simulink model "foc"  (R2021b)
settings: Solver=FixedStepDiscrete  StartTime=0.0  StopTime=20  FixedStep=Ts  MaxStep=1e-4  RelTol=1e-3
model workspace (MAT data in the model file):
  flux = 0.154
values from neighbouring files (symbols this model uses):
  currt_width = 200.0    [motor_parameters.sldd]
  Flux = 0.00103001    [motor_parameters.sldd]
  Ibus = 5.0    [motor_parameters.sldd]
  Ld = 2.235E-5    [motor_parameters.sldd]
  Lq = 2.567E-5    [motor_parameters.sldd]
  Ls = 2.235E-5    [motor_parameters.sldd]
  OPL_time = 3.0    [motor_parameters.sldd]
  Pn = 7.0    [motor_parameters.sldd]
  R = 0.083    [motor_parameters.sldd]
  Rs = 0.112    [motor_parameters.sldd]
  smo_l = 0.1    [motor_parameters.sldd]
  smo_m = 0.001    [motor_parameters.sldd]
  Ts = 0.0001    [motor_parameters.sldd]
  Ubus = 12.0    [motor_parameters.sldd]
undefined symbols (not defined in the file or in its folder): DiscIntNeverNeededParam, sigbuilder_block, spd_ki, spd_kp
libraries: slpidlib x5, simulink x3, mcbcontrolslib x3, mcbplantlib x1, autolibpmsmexterior x1
(part 1 of 2)
settings Model: DataDictionary=motor_parameters.sldd  Creator=chenpeng  LastModifiedBy=chenpeng
settings OptimizationCC: DefaultParameterBehavior=Inlined  UseDivisionForNetSlopeComputation=on  GainParamInheritBuiltInType=on  UseFloatMulNetSlope=on  InlineInvariantSignals=on  PassReuseOutputArgsAs=Individual arguments  ZeroExternalMemoryAtStartup=off  ZeroInternalMemoryAtStartup=off  NoFixptDivByZeroProtection=on  EfficientFloat2IntCast=on  LifeSpan=1  OptimizeBlockOrder=speed  DifferentSizesBufferReuse=on  EfficientTunableParamExpr=on
settings DebuggingCC: AlgebraicLoopMsg=none  ParameterTunabilityLossMsg=error
settings HardwareCC: ProdBitPerPointer=32  ProdBitPerSizeT=32  ProdBitPerPtrDiffT=32  ProdLargestAtomicInteger=Long  ProdLargestAtomicFloat=Double  ProdWordSize=32  ProdLongLongMode=on  ProdHWDeviceType=ARM Compatible->ARM Cortex-M
settings SFSimCC: MATLABDynamicMemAlloc=off
settings RTWCC: Description=Embedded Coder  SystemTargetFile=ert.tlc  GenCodeOnly=on  TemplateMakefile=ert_default_tmf  Toolchain=GNU Tools for ARM Embedded Processors
settings CodeAppCC: ForceParamTrailComments=on  IgnoreCustomStorageClasses=off  OperatorAnnotations=on  SimulinkDataObjDesc=on  SFDataObjDesc=on  CustomSymbolStrGlobalVar=rt$N$M  CustomSymbolStrType=$N$M  CustomSymbolStrFcn=$N$M$F  CustomSymbolStrMacro=$N$M  InsertBlockDesc=on
settings ERTTargetCC: TargetLangStandard=C99 (ISO)  GenerateSampleERTMain=on  IncludeMdlTerminateFcn=off  CombineSignalStateStructs=on  SupportComplex=off  SupportNonInlinedSFcns=on  InlinedParameterPlacement=NonHierarchical  ERTCustomFileTemplate=example_file_process.tlc  ERTFilePackagingFormat=CompactWithDataFile

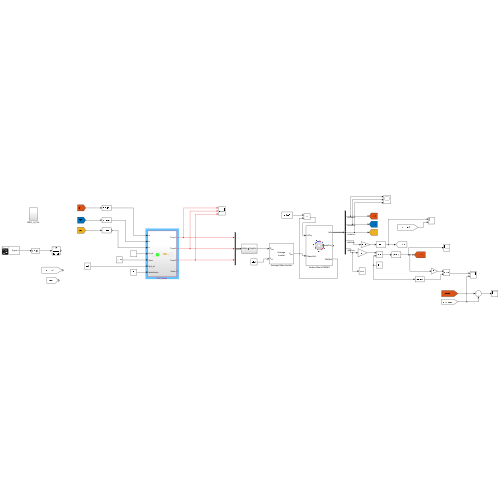
[thumbnail: Simulink's stored preview of the top-level diagram]
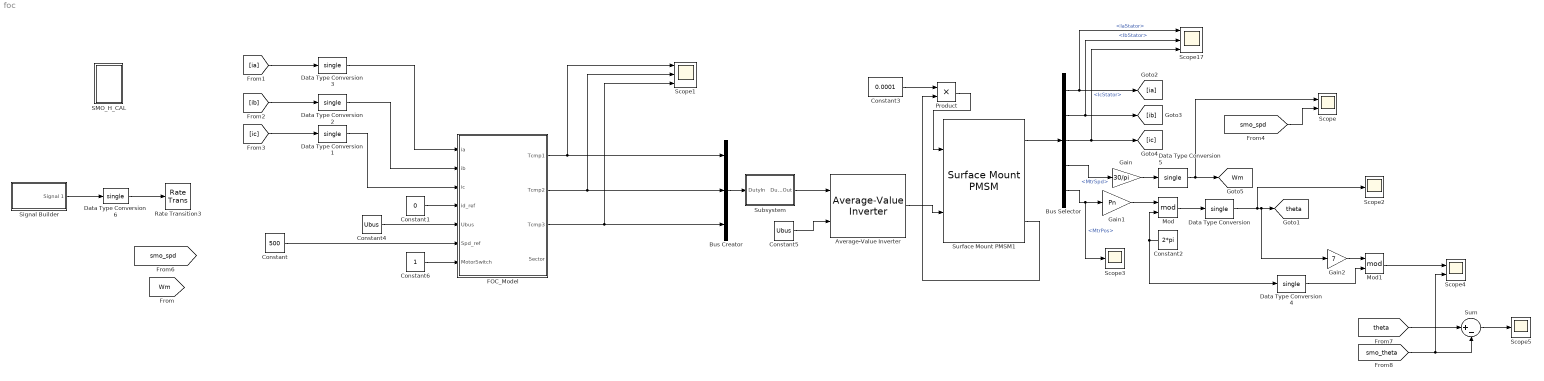
== system foc ==
  Average-Value Inverter : mcbplantlib/Average-Value Inverter
  Bus Creator : BusCreator  Inputs=3
  Bus Selector : BusSelector  OutputSignals=IaStator,IbStator,IcStator,MtrSpd,MtrPos
  Constant : Constant  Value=500  OutDataTypeStr=single  SampleTime=-1
  Constant1 : Constant  Value=0  OutDataTypeStr=single  SampleTime=-1
  Constant2 : Constant  Value=2*pi
  Constant3 : Constant  Value=0.0001  OutDataTypeStr=double
  Constant4 : Constant  Value=Ubus  OutDataTypeStr=single
  Constant5 : Constant  Value=Ubus  OutDataTypeStr=single
  Constant6 : Constant  OutDataTypeStr=single  SampleTime=-1
  Data Type Conversion{,1..6} (7 alike) : DataTypeConversion  OutDataTypeStr=single
  FOC_Model : Subsystem
  Gain : Gain  Gain=30/pi
  Gain1 : Gain  Gain=Pn
  Gain2 : Gain  Gain=7
  Mod : Math  Operator=mod  SaturateOnIntegerOverflow=on
  Mod1 : Math  Operator=mod  SaturateOnIntegerOverflow=on
  Product : Product
  Rate Transition3 : RateTransition
  SMO_H_CAL : Subsystem
  Scope : Scope  NumInputPorts=2
  Scope1 : Scope  NumInputPorts=3
  Scope17 : Scope  NumInputPorts=3
  Scope2 : Scope
  Scope3 : Scope
  Scope4 : Scope  NumInputPorts=2
  Scope5 : Scope
  Signal Builder : Subsystem  Tag=STV Subsys  LoadFcn=sigbuilder_block('load');  StartFcn=sigbuilder_block('start');  StopFcn=sigbuilder_block('stop');  ClipboardFcn=sigbuilder_block('clipboard');  mask(Sigbuilder block){tuvar=[0:10]}
      mask help: Simulink:masks:SigbuilderBlock_MD
      mask init:
      | if ~strcmp(get_param(bdroot(gcbh),'SimulationStatus'),'stopped') tuvar = sigbuilder_block('maskInit'); end
      settings: CopyFcn=sigbuilder_block('copy');  DeleteFcn=sigbuilder_block('delete');  ModelCloseFcn=sigbuilder_block('modelClose');  PreSaveFcn=sigbuilder_block('preSave');  PauseFcn=sigbuilder_block('pause');  ContinueFcn=sigbuilder_block('continue');  NameChangeFcn=sigbuilder_block('namechange');  OpenFcn=sigbuilder_block('open',[437.6 199.2 550.4 400 ]);  CloseFcn=sigbuilder_block('close');
      mask Display: plot(0, 0, 100, 100,[2, 2, 32, 32, 2], [68, 8, 8, 68, 68],[32, 2], [38, 38], [32, 19, 2],[53, 60, 44], [32, 17, 17, 2],[16, 16, 31, 31]);txt = getActiveGroup(gcbh);text(2, 100, txt,'verticalAlignment', 'top');
  Subsystem : Subsystem
  Sum : Sum  Inputs=|+-
  Surface Mount PMSM1 : autolibpmsmexterior/Surface Mount PMSM  port_config=Torque  sim_type=Discrete  Ts=Ts  FilePath=E:\Sandbox\Bauto\Work\surfacepmsm_motordata.m  P=Pn  Rs=Rs  Ldq_=Ls  KConstText=Permanent flux linkage constant (lambda_pm):  lambda_pm=Flux  Ke=159.9771  Kt=1.323  mechanical=[0.0027, 4.924e-4, 0]  idq0=[0 0]  theta_init=0  omega_init=0  KConst=Flux  lambda_pm_calc=Flux  RefBlkName='autolibpmsmexterior/Surface Mount PMSM'  aMode=1  Ldq="[0.0003752   0.0003752]"
      settings: SourceProductBaseCode=PW,DR,MT,UV,VE
  tag scope: Wm=global, theta=global
  wires:
  Data Type Conversion/1 -> Scope2/1, Gain2/1, [theta]
  Bus Selector/3 -> Scope17/3, [ic]  "<IcStator>"
  Mod/1 -> Data Type Conversion/1
  Gain/1 -> Data Type Conversion5/1
  Constant3/1 -> Product/1
  Gain1/1 -> Mod/1
  Data Type Conversion5/1 -> Scope/1, [Wm]
  Bus Creator/1 -> Subsystem/1(DutyIn)
  Bus Selector/5 -> Scope3/1, Gain1/1  "<MtrPos>"
  Bus Selector/1 -> [ia], Scope17/1  "<IaStator>"
  Subsystem/1(DutyOut) -> Average-Value Inverter/1
  Bus Selector/2 -> Scope17/2, [ib]  "<IbStator>"
  Bus Selector/4 -> Gain/1  "<MtrSpd>"
  Constant2/1 -> Data Type Conversion4/1, Mod/2
  Constant5/1 -> Average-Value Inverter/2
  [ia] -> Data Type Conversion3/1
  [ib] -> Data Type Conversion2/1
  [ic] -> Data Type Conversion1/1
  Average-Value Inverter/1 -> Surface Mount PMSM1/2
  Surface Mount PMSM1/3 -> Product/2
  Surface Mount PMSM1/1 -> Bus Selector/1
  Gain2/1 -> Mod1/1
  Mod1/1 -> Scope4/1
  Data Type Conversion4/1 -> Mod1/2
  Product/1 -> Surface Mount PMSM1/1
  Data Type Conversion3/1 -> FOC_Model/1(ia)
  Data Type Conversion2/1 -> FOC_Model/2(ib)
  Data Type Conversion1/1 -> FOC_Model/3(ic)
  Constant4/1 -> FOC_Model/5(Ubus)
  FOC_Model/1(Tcmp1) -> Scope1/1, Bus Creator/1
  FOC_Model/2(Tcmp2) -> Scope1/2, Bus Creator/2
  FOC_Model/3(Tcmp3) -> Scope1/3, Bus Creator/3
  Constant6/1 -> FOC_Model/7(MotorSwitch)
  [smo_spd] -> Scope/2
  Constant1/1 -> FOC_Model/4(id_ref)
  [smo_theta] -> Scope4/2, Sum/2
  Sum/1 -> Scope5/1
  Data Type Conversion6/1 -> Rate Transition3/1
  Signal Builder/1(Signal 1) -> Data Type Conversion6/1
  Constant/1 -> FOC_Model/6(Spd_ref)
  [theta] -> Sum/1

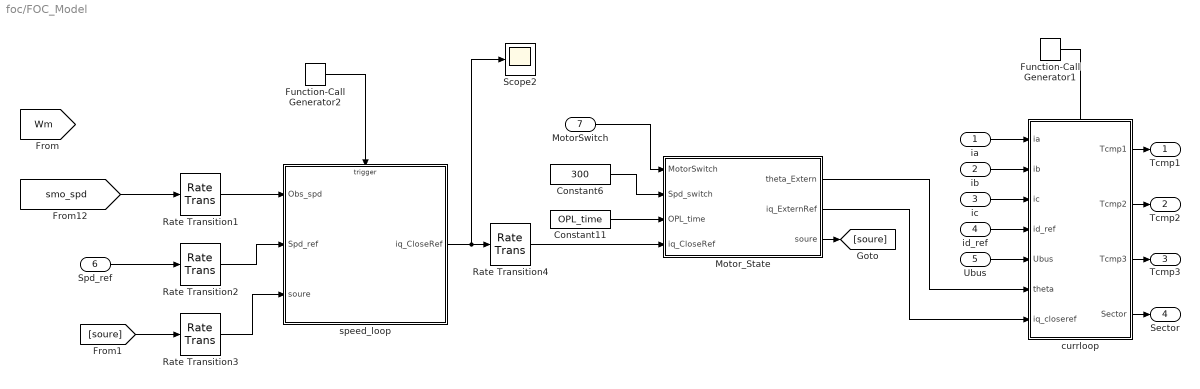
== system foc/FOC_Model ==
  ia : Inport  OutDataTypeStr=single
  ib : Inport  Port=2  OutDataTypeStr=single
  ic : Inport  Port=3  OutDataTypeStr=single
  id_ref : Inport  Port=4  OutDataTypeStr=single
  Ubus : Inport  Port=5  OutDataTypeStr=single
  Spd_ref : Inport  Port=6  OutDataTypeStr=single
  MotorSwitch : Inport  Port=7  OutDataTypeStr=single
  Constant11 : Constant  Value=OPL_time  OutDataTypeStr=single
  Constant6 : Constant  Value=300  OutDataTypeStr=int32
  Function-Call Generator1 : simulink/Ports & Subsystems/Function-Call Generator  sample_time=1e-4  numberOfIterations=1  DisallowWideOutput=off
  Function-Call Generator2 : simulink/Ports & Subsystems/Function-Call Generator  sample_time=1e-3  numberOfIterations=1  DisallowWideOutput=off
  Motor_State : Subsystem
  Rate Transition{1..4} (4 alike) : RateTransition
  Scope2 : Scope
  currloop : Subsystem
  speed_loop : Subsystem  TreatAsAtomicUnit=on  SystemSampleTime=1e-4
      settings: RTWSystemCode=Nonreusable function  RTWFcnNameOpts=Use subsystem name
  Tcmp1 : Outport  OutDataTypeStr=single
  Tcmp2 : Outport  Port=2  OutDataTypeStr=single
  Tcmp3 : Outport  Port=3  OutDataTypeStr=single
  Sector : Outport  Port=4  OutDataTypeStr=single
  wires:
  Rate Transition1/1 -> speed_loop/1(Obs_spd)
  ia/1 -> currloop/1(ia)
  ib/1 -> currloop/2(ib)
  Ubus/1 -> currloop/5(Ubus)
  currloop/4(Sector) -> Sector/1
  currloop/2(Tcmp2) -> Tcmp2/1
  Rate Transition2/1 -> speed_loop/2(Spd_ref)
  speed_loop/1(iq_CloseRef) -> Scope2/1, Rate Transition4/1
  ic/1 -> currloop/3(ic)
  id_ref/1 -> currloop/4(id_ref)
  currloop/1(Tcmp1) -> Tcmp1/1
  currloop/3(Tcmp3) -> Tcmp3/1
  Spd_ref/1 -> Rate Transition2/1
  Constant11/1 -> Motor_State/3(OPL_time)
  Rate Transition4/1 -> Motor_State/4(iq_CloseRef)
  Constant6/1 -> Motor_State/2(Spd_switch)
  MotorSwitch/1 -> Motor_State/1(MotorSwitch)
  Motor_State/1(theta_Extern) -> currloop/6(theta)
  Motor_State/2(iq_ExternRef) -> currloop/7(iq_closeref)
  Function-Call Generator1/1 -> ?
  Rate Transition3/1 -> speed_loop/3(soure)
  Function-Call Generator2/1 -> speed_loop/Trigger
  Motor_State/3(soure) -> [soure]
  [soure] -> Rate Transition3/1
  [smo_spd] -> Rate Transition1/1

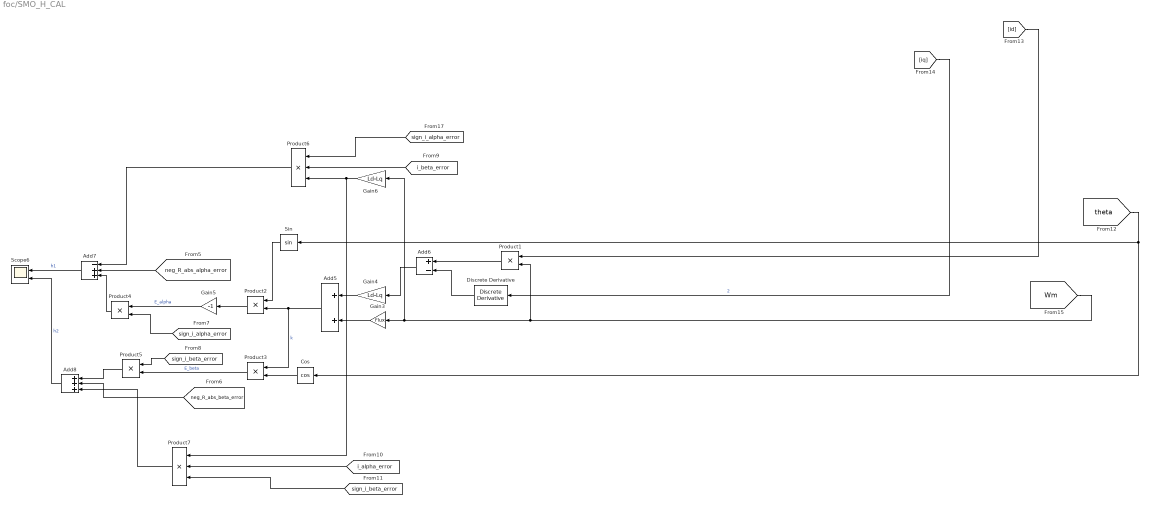
== system foc/SMO_H_CAL ==
  Add5 : Sum
  Add6 : Sum  Inputs=+-
  Add7 : Sum  Inputs=-++  AccumDataTypeStr=single
  Add8 : Sum  Inputs=+++
  Cos : Trigonometry  Operator=cos
  Discrete Derivative : simulink/Discrete/Discrete Derivative  gainval=1.0  ICPrevScaledInput=0.0  OutMin=[]  OutMax=[]  OutDataType=fixdt(1, 16)  OutScaling=2^-10  DoSatur=off
  Gain3 : Gain  Gain=Flux
  Gain4 : Gain  Gain=Ld-Lq
  Gain5 : Gain  Gain=-1
  Gain6 : Gain  Gain=Ld-Lq
  Product{1..5} (5 alike) : Product
  Product6 : Product  Inputs=3  OutDataTypeStr=single
  Product7 : Product  Inputs=3
  Scope6 : Scope  NumInputPorts=2
  Sin : Trigonometry
  wires:
  Add5/1 -> Product3/1, Product2/2  "k"
  [sign_i_beta_error] -> Product7/3
  Cos/1 -> Product3/2
  [neg_R_abs_beta_error] -> Add8/2
  Gain6/1 -> Product6/3, Product7/1
  [sign_i_alpha_error] -> Product4/2
  [theta] -> Cos/1, Sin/1
  [iq] -> Discrete Derivative/1  "2"
  Product1/1 -> Add6/1
  [Wm] -> Gain6/1, Gain3/1, Product1/2
  [sign_i_alpha_error] -> Product6/1
  Product6/1 -> Add7/1
  [neg_R_abs_alpha_error] -> Add7/2
  Product4/1 -> Add7/3
  Product2/1 -> Gain5/1
  [i_alpha_error] -> Product7/2
  Gain4/1 -> Add5/1
  Discrete Derivative/1 -> Add6/2
  Add7/1 -> Scope6/1  "h1"
  [id] -> Product1/1
  [i_beta_error] -> Product6/2
  Gain5/1 -> Product4/1  "E_alpha"
  Product3/1 -> Product5/2  "E_beta"
  Product7/1 -> Add8/3
  Add6/1 -> Gain4/1
  Add8/1 -> Scope6/2  "h2"
  Gain3/1 -> Add5/2
  [sign_i_beta_error] -> Product5/1
  Sin/1 -> Product2/1
  Product5/1 -> Add8/1

== system foc/Signal Builder ==
  Demux : Demux  Tag=STV Demux  Outputs=1
      settings: DisplayOption=none
  FromWs : FromWorkspace  Tag=STV FromWs  VariableName=tuvar
      SigBuilderData=|
      | common.afterFinalStr = 'Extrapolate'
      | common.sampleTime = 0
      | dataSet.timeRange = [0 10]
      | dataSet.name = 'Group 1'
      | sbobj.Groups.Name = 'Group 1'
      | sbobj.Groups.Signals.Name = 'Signal 1'
      | sbobj.Groups.Signals.XData = [0 4 4 7 7 10]
      | sbobj.Groups.Signals.YData = [400 395 598 602 800 802]
  Signal 1 : Outport  Tag=STV Outport
  wires:
  Demux/1 -> Signal 1/1
  FromWs/1 -> Demux/1

== system foc/Subsystem ==
  DutyIn : Inport
  Constant : Constant  Value=0.5  OutDataTypeStr=double  SampleTime=-1
  Gain : Gain  Gain=1/8000  ParamDataTypeStr=single
  Gain1 : Gain  Gain=-1
  Sum : Sum  Inputs=|+-
  Sum1 : Sum  Inputs=|++
  DutyOut : Outport
  wires:
  Sum/1 -> Gain1/1
  Constant/1 -> Sum1/2, Sum/2
  DutyIn/1 -> Gain/1
  Gain1/1 -> Sum1/1
  Sum1/1 -> DutyOut/1
  Gain/1 -> Sum/1

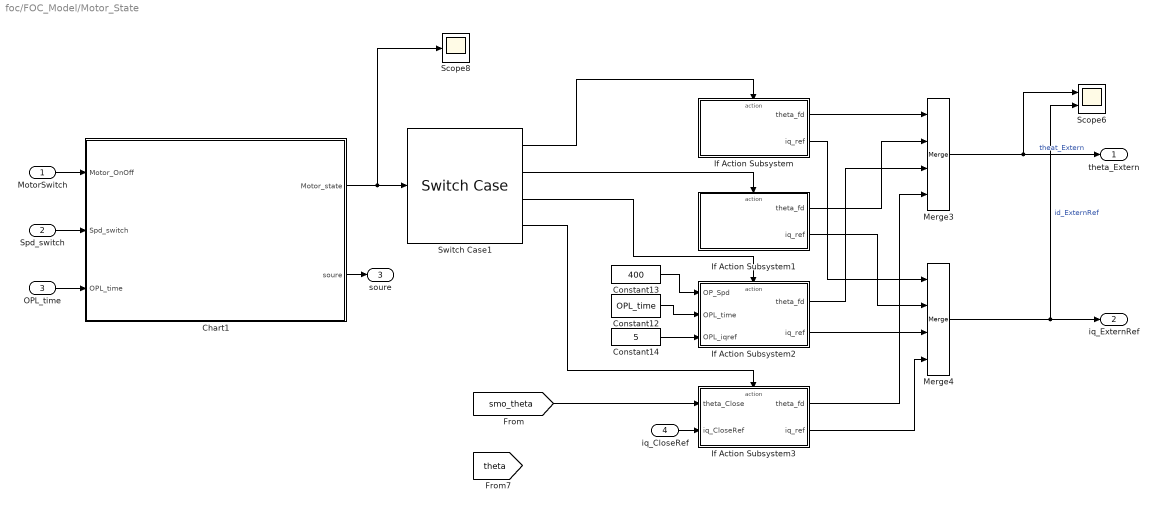
== system foc/FOC_Model/Motor_State ==
  MotorSwitch : Inport
  Spd_switch : Inport  Port=2  OutDataTypeStr=int32
  OPL_time : Inport  Port=3  OutDataTypeStr=single
  iq_CloseRef : Inport  Port=4
  Chart1 : Stateflow chart  TreatAsAtomicUnit=on
  Constant12 : Constant  Value=OPL_time  OutDataTypeStr=single
  Constant13 : Constant  Value=400  OutDataTypeStr=int32
  Constant14 : Constant  Value=5  OutDataTypeStr=single
  If Action Subsystem : Subsystem  TreatAsAtomicUnit=on
  If Action Subsystem1 : Subsystem  TreatAsAtomicUnit=on
  If Action Subsystem2 : Subsystem  TreatAsAtomicUnit=on
  If Action Subsystem3 : Subsystem  TreatAsAtomicUnit=on
  Merge3 : Merge  Inputs=4
  Merge4 : Merge  Inputs=4
  Scope6 : Scope  NumInputPorts=2
  Scope8 : Scope
  Switch Case1 : SwitchCase  CaseConditions={1,2,3,4}  ShowDefaultCase=off
  theta_Extern : Outport  OutDataTypeStr=single
  iq_ExternRef : Outport  Port=2  OutDataTypeStr=single
  soure : Outport  Port=3
  wires:
  Constant13/1 -> If Action Subsystem2/1(OP_Spd)
  Constant14/1 -> If Action Subsystem2/3(OPL_iqref)
  Constant12/1 -> If Action Subsystem2/2(OPL_time)
  iq_CloseRef/1 -> If Action Subsystem3/2(iq_CloseRef)
  Switch Case1/4 -> If Action Subsystem3/Action
  If Action Subsystem/1(theta_fd) -> Merge3/1
  Chart1/2(soure) -> soure/1
  OPL_time/1 -> Chart1/3(OPL_time)
  Merge4/1 -> iq_ExternRef/1, Scope6/2  "id_ExternRef"
  Spd_switch/1 -> Chart1/2(Spd_switch)
  Merge3/1 -> Scope6/1, theta_Extern/1  "theat_Extern"
  If Action Subsystem1/2(iq_ref) -> Merge4/2
  Chart1/1(Motor_state) -> Switch Case1/1, Scope8/1
  If Action Subsystem/2(iq_ref) -> Merge4/1
  Switch Case1/2 -> If Action Subsystem1/Action
  Switch Case1/1 -> If Action Subsystem/Action
  If Action Subsystem3/1(theta_fd) -> Merge3/4
  Switch Case1/3 -> If Action Subsystem2/Action
  If Action Subsystem2/2(iq_ref) -> Merge4/3
  If Action Subsystem3/2(iq_ref) -> Merge4/4
  MotorSwitch/1 -> Chart1/1(Motor_OnOff)
  If Action Subsystem2/1(theta_fd) -> Merge3/3
  If Action Subsystem1/1(theta_fd) -> Merge3/2
  [smo_theta] -> If Action Subsystem3/1(theta_Close)

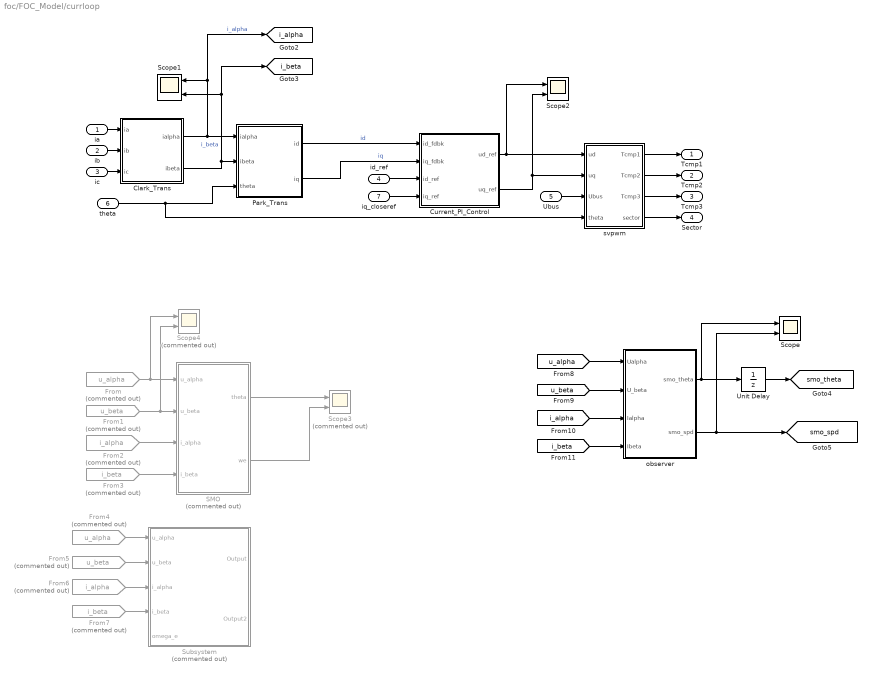
== system foc/FOC_Model/currloop ==
  ia : Inport  OutDataTypeStr=single  SampleTime=0.0001
  ib : Inport  Port=2  OutDataTypeStr=single  SampleTime=0.0001
  ic : Inport  Port=3  OutDataTypeStr=single  SampleTime=0.0001
  id_ref : Inport  Port=4  OutDataTypeStr=single  SampleTime=0.0001
  Ubus : Inport  Port=5  SampleTime=0.0001
  theta : Inport  Port=6  OutDataTypeStr=single  SampleTime=0.0001
  iq_closeref : Inport  Port=7  OutDataTypeStr=single  SampleTime=0.0001
  Clark_Trans : Subsystem  TreatAsAtomicUnit=on
  Current_PI_Control : Subsystem
  From : From  Commented=on  GotoTag=u_alpha  TagVisibility=global
  From1 : From  Commented=on  GotoTag=u_beta  TagVisibility=global
  From2 : From  Commented=on  GotoTag=i_alpha  TagVisibility=global
  From3 : From  Commented=on  GotoTag=i_beta  TagVisibility=global
  From4 : From  Commented=on  GotoTag=u_alpha  TagVisibility=global
  From5 : From  Commented=on  GotoTag=u_beta  TagVisibility=global
  From6 : From  Commented=on  GotoTag=i_alpha  TagVisibility=global
  From7 : From  Commented=on  GotoTag=i_beta  TagVisibility=global
  Park_Trans : Subsystem  TreatAsAtomicUnit=on
  SMO : Subsystem  Commented=on
      settings: PortSchema="{\"entries\":[{\"content\":{\"sides\":[{\"content\":{\"connectorIds\":[\"Out1\",\"Out2\"]},\"type\":\"ConnectorPlacement.EquallySpacedRectSide\",\"uuid\":\"5414e755-aa17-4597-a468-b801bf68950d\"},{\"content\":{\"connectorIds\":[\"In1\",\"In2\",\"In3\",\"In4\"],\"side\":\"RIGHT\"},\"type\":\"ConnectorPlacement.EquallySpacedRectSide\",\"uuid\":\"33e6150f-a627-4b89-8f54-9d41cb10a0e9\"},{\"content\":{\"connectorIds\":[],\"side\":\"TOP\"},\"type\":\"ConnectorPlacement.EquallySpacedRectSide\",\"uuid\":\"8ba45070-0913-41de-bd30-b153cef900e1\"}]},\"type\":\"ConnectorPlacement.EquallySpacedConnector\",\"uuid\":\"5336ec09-c709-45c9-9606-7ae9e0652068\"}],\"packageUris\":[\"http://schema.mathworks.com/mf0/Connector/R2020b\"],\"version\":\"1.0\"}"
  Scope : Scope  NumInputPorts=2
  Scope1 : Scope  NumInputPorts=2
  Scope2 : Scope  NumInputPorts=2
  Scope3 : Scope  Commented=on  NumInputPorts=2
  Scope4 : Scope  Commented=on  NumInputPorts=2
  Subsystem : Subsystem  Commented=on
  Unit Delay : UnitDelay  SampleTime=-1  HasFrameUpgradeWarning=on
  observer : Subsystem
  svpwm : Subsystem
  Tcmp1 : Outport
  Tcmp2 : Outport  Port=2
  Tcmp3 : Outport  Port=3
  Sector : Outport  Port=4
  tag scope: i_alpha=global, i_beta=global, smo_spd=global, smo_theta=global
  wires:
  Park_Trans/2(iq) -> Current_PI_Control/2(iq_fdbk)  "iq"
  ia/1 -> Clark_Trans/1(ia)
  ic/1 -> Clark_Trans/3(ic)
  Park_Trans/1(id) -> Current_PI_Control/1(id_fdbk)  "id"
  ib/1 -> Clark_Trans/2(ib)
  Current_PI_Control/1(ud_ref) -> Scope2/1, svpwm/1(ud)
  Current_PI_Control/2(uq_ref) -> Scope2/2, svpwm/2(uq)
  svpwm/1(Tcmp1) -> Tcmp1/1
  svpwm/2(Tcmp2) -> Tcmp2/1
  svpwm/3(Tcmp3) -> Tcmp3/1
  svpwm/4(sector) -> Sector/1
  Ubus/1 -> svpwm/3(Ubus)
  id_ref/1 -> Current_PI_Control/3(id_ref)
  From/1 -> Scope4/1, SMO/1(u_alpha)
  From1/1 -> Scope4/2, SMO/2(u_beta)
  From2/1 -> SMO/3(i_alpha)
  From3/1 -> SMO/4(i_beta)
  SMO/1(theta) -> Scope3/1
  SMO/2(we) -> Scope3/2
  Clark_Trans/2(ibeta) -> [i_beta], Scope1/2, Park_Trans/2(ibeta)  "i_beta"
  Clark_Trans/1(ialpha) -> [i_alpha], Scope1/1, Park_Trans/1(ialpha)  "i_alpha"
  From4/1 -> Subsystem/1(u_alpha)
  From7/1 -> Subsystem/4(i_beta)
  From6/1 -> Subsystem/3(i_alpha)
  From5/1 -> Subsystem/2(u_beta)
  theta/1 -> svpwm/4(theta), Park_Trans/3(theta)
  iq_closeref/1 -> Current_PI_Control/4(iq_ref)
  [u_alpha] -> observer/1(Ualpha)
  observer/1(smo_theta) -> Unit Delay/1, Scope/1
  observer/2(smo_spd) -> [smo_spd], Scope/2
  [i_beta] -> observer/4(Ibeta)
  [u_beta] -> observer/2(U_beta)
  [i_alpha] -> observer/3(Ialpha)
  Unit Delay/1 -> [smo_theta]

== system foc/FOC_Model/speed_loop ==
  Obs_spd : Inport  OutDataTypeStr=single  PortDimensions=1
  Spd_ref : Inport  Port=2  OutDataTypeStr=single  PortDimensions=1
  soure : Inport  Port=3  OutDataTypeStr=single  PortDimensions=1
  Trigger : TriggerPort  TriggerType=function-call  VariantControl=(inherit)  PortDimensions=1
  Constant : Constant  Value=0.0144  OutDataTypeStr=single  SampleTime=-1
  Constant1 : Constant  Value=0.6389  OutDataTypeStr=single  SampleTime=-1
  PID Controller3 : slpidlib/PID Controller  Controller=PI  Form=Parallel  TimeDomain=Discrete-time  UseExternalTs=off  SampleTime=-1  IntegratorMethod=Forward Euler  FilterMethod=Forward Euler  ControllerParametersSource=external  P=spd_kp  I=spd_ki  D=0  UseFilter=on  N=100  TunerSelectOption=Transfer Function Based (PID Tuner App)  InitialConditionSource=internal  InitialConditionForIntegrator=0  InitialConditionForFilter=0  DifferentiatorICPrevScaledInput=0  ExternalReset=rising  TrackingMode=off  Kt=1  LimitOutput=on  SatLimitsSource=internal  UpperSaturationLimit=Ibus  LowerSaturationLimit=-Ibus  LinearizeAsGain=on  AntiWindupMode=clamping  Kb=0.013  PGainOutDataTypeStr=single  PProdOutDataTypeStr=single  POutMin=[]  POutMax=[]  IGainOutDataTypeStr=single  IProdOutDataTypeStr=single  IOutMin=[]  IOutMax=[]  DOutMin=[]  DOutMax=[]  NOutMin=[]  NOutMax=[]  SumOutDataTypeStr=single  SumOutMin=[]  SumOutMax=[]  SaturationOutDataTypeStr=single  SaturationOutMin=[]  SaturationOutMax=[]  PParamMin=[]  PParamMax=[]  IParamMin=[]  IParamMax=[]  DParamMin=[]  DParamMax=[]  NParamMin=[]  NParamMax=[]  KbParamMin=[]  KbParamMax=[]  KtParamMin=[]  KtParamMax=[]  KbOutMin=[]  KbOutMax=[]  KtOutMin=[]  KtOutMax=[]  IntegratorOutMin=[]  IntegratorOutMax=[]  FilterOutMin=[]  FilterOutMax=[]  SumI1OutMin=[]  SumI1OutMax=[]  SumI2OutMin=[]  SumI2OutMax=[]  SumI3OutMin=[]  SumI3OutMax=[]  SumI4OutMin=[]  SumI4OutMax=[]  SumDOutMin=[]  SumDOutMax=[]  DifferentiatorOutMin=[]  DifferentiatorOutMax=[]  FilterDiffOutCoefMin=[]  FilterDiffOutCoefMax=[]  ReciprocalOutMin=[]  ReciprocalOutMax=[]  SumDenOutMin=[]  SumDenOutMax=[]  SumNumOutMin=[]  SumNumOutMax=[]  DivideOutMin=[]  DivideOutMax=[]  UdiffTsProdOutMin=[]  UdiffTsProdOutMax=[]  NTsProdOutMin=[]  NTsProdOutMax=[]  UintegralTsProdOutMin=[]  UintegralTsProdOutMax=[]  UngainTsProdOutMin=[]  UngainTsProdOutMax=[]  IntegratorContinuousStateAttributes=''  IntegratorStateMustResolveToSignalObject=off  IntegratorRTWStateStorageClass=Auto  FilterContinuousStateAttributes=''  FilterStateMustResolveToSignalObject=off  FilterRTWStateStorageClass=Auto  ParallelPVariant=ExternalParameters  IdealPVariant=Disabled  IVariant=ExternalParameters  DVariant=Disabled  IntegratorVariant=Discrete  SatVariant=Enabled  AWVariant=DiscClampingParallel  PCopyVariant=Disabled  TRVariant=Disabled  FdbkBlocksVariant=Forward  IdealPFdbkVariant=Disabled  SatFdbkVariant=Disabled  DerivativeFilterVariant=Disabled  NVariant=Disabled  NCopyVariant=Disabled_SignalSpec  FilterICVariant=Disabled  IntegratorICVariant=InternalICs  ExternalResetVariant=ExternalReset  TRSumVariant=Passthrough  SumFdbkVariant=Disabled  SumVariant=Sum_PI  TsampFilterVariant=InternalTs  TsampNgainVariant=Passthrough  TsampIntegralVariant=Passthrough  ExternalSaturationOutDataTypeStr=single
  Scope : Scope
  Sum2 : Sum  Inputs=|+-  AccumDataTypeStr=single  OutDataTypeStr=single
  iq_CloseRef : Outport
  wires:
  Obs_spd/1 -> Sum2/2
  Spd_ref/1 -> Sum2/1
  Sum2/1 -> Scope/1, PID Controller3/1
  PID Controller3/1 -> iq_CloseRef/1
  Constant/1 -> PID Controller3/2
  Constant1/1 -> PID Controller3/3
  soure/1 -> PID Controller3/4

== system foc/FOC_Model/Motor_State/If Action Subsystem ==
  Action Port : ActionPort  ActionPortLabel=case [ 1 ]:
  Constant : Constant  Value=0  OutDataTypeStr=single  SampleTime=-1
  Constant1 : Constant  Value=0  OutDataTypeStr=single  SampleTime=-1
  theta_fd : Outport
  iq_ref : Outport  Port=2
  wires:
  Constant/1 -> theta_fd/1
  Constant1/1 -> iq_ref/1

== system foc/FOC_Model/Motor_State/If Action Subsystem1 ==
  Action Port : ActionPort  ActionPortLabel=case [ 2 ]:
  Constant : Constant  Value=0  OutDataTypeStr=single  SampleTime=-1
  Constant1 : Constant  Value=2  OutDataTypeStr=single  SampleTime=-1
  theta_fd : Outport
  iq_ref : Outport  Port=2
  wires:
  Constant/1 -> theta_fd/1
  Constant1/1 -> iq_ref/1

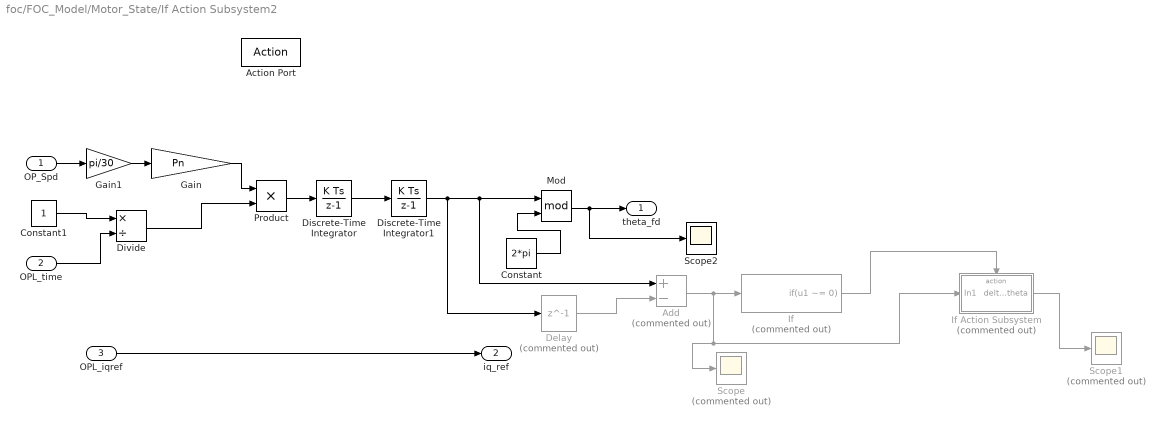
== system foc/FOC_Model/Motor_State/If Action Subsystem2 ==
  OP_Spd : Inport  OutDataTypeStr=int32  PortDimensions=1
  OPL_time : Inport  Port=2  OutDataTypeStr=single  PortDimensions=1
  OPL_iqref : Inport  Port=3  OutDataTypeStr=single  PortDimensions=1
  Action Port : ActionPort  ActionPortLabel=case [ 3 ]:
  Add : Sum  Commented=on  Inputs=+-  AccumDataTypeStr=single  OutDataTypeStr=single
  Constant : Constant  Value=2*pi  OutDataTypeStr=single  SampleTime=-1
  Constant1 : Constant  OutDataTypeStr=single  SampleTime=-1
  Delay : Delay  Commented=on  DelayLength=1  InputProcessing=Columns as channels (frame based)
  Discrete-Time Integrator : DiscreteIntegrator  SampleTime=-1  ICPrevOutput=DiscIntNeverNeededParam  ICPrevScaledInput=DiscIntNeverNeededParam
  Discrete-Time Integrator1 : DiscreteIntegrator  SampleTime=-1  ICPrevOutput=DiscIntNeverNeededParam  ICPrevScaledInput=DiscIntNeverNeededParam
  Divide : Product  Inputs=*/  OutDataTypeStr=single
  Gain : Gain  Gain=Pn
  Gain1 : Gain  Gain=pi/30  OutDataTypeStr=single
  If : If  Commented=on  IfExpression=u1 ~= 0  ShowElse=off
  If Action Subsystem : Subsystem  Commented=on  TreatAsAtomicUnit=on
  Mod : Math  Operator=mod  SaturateOnIntegerOverflow=on
  Product : Product  OutDataTypeStr=single
  Scope : Scope  Commented=on
  Scope1 : Scope  Commented=on
  Scope2 : Scope
  theta_fd : Outport
  iq_ref : Outport  Port=2
  wires:
  Gain1/1 -> Gain/1
  Constant1/1 -> Divide/1
  Gain/1 -> Product/1
  Discrete-Time Integrator/1 -> Discrete-Time Integrator1/1
  Constant/1 -> Mod/2
  Discrete-Time Integrator1/1 -> Delay/1, Add/1, Mod/1
  Mod/1 -> Scope2/1, theta_fd/1
  OPL_time/1 -> Divide/2
  OPL_iqref/1 -> iq_ref/1
  Divide/1 -> Product/2
  Product/1 -> Discrete-Time Integrator/1
  OP_Spd/1 -> Gain1/1
  Delay/1 -> Add/2
  Add/1 -> If Action Subsystem/1(In1), Scope/1, If/1
  If/1 -> If Action Subsystem/Action
  If Action Subsystem/1(delta_theta) -> Scope1/1

== system foc/FOC_Model/Motor_State/If Action Subsystem3 ==
  theta_Close : Inport
  iq_CloseRef : Inport  Port=2
  Action Port : ActionPort  ActionPortLabel=case [ 4 ]:
  theta_fd : Outport
  iq_ref : Outport  Port=2
  wires:
  theta_Close/1 -> theta_fd/1
  iq_CloseRef/1 -> iq_ref/1

== system foc/FOC_Model/currloop/Clark_Trans ==
  note: ialpha = ia*2/3-(ib+ic)/3;
      | ibeta = (ib-ic)*sqrt(3)/3;
  ia : Inport  OutDataTypeStr=single
  ib : Inport  Port=2  OutDataTypeStr=single
  ic : Inport  Port=3  OutDataTypeStr=single
  Add : Sum  AccumDataTypeStr=single  OutDataTypeStr=single
  Add1 : Sum  Inputs=+-  AccumDataTypeStr=single  OutDataTypeStr=single
  Add2 : Sum  Inputs=+-  AccumDataTypeStr=single  OutDataTypeStr=single
  Gain : Gain  Gain=2/3  ParamDataTypeStr=single
  Gain1 : Gain  Gain=1/3  ParamDataTypeStr=single
  Gain2 : Gain  Gain=sqrt(3)/3  ParamDataTypeStr=single
  ialpha : Outport  OutDataTypeStr=single
  ibeta : Outport  Port=2  OutDataTypeStr=single
  wires:
  ia/1 -> Gain/1
  ib/1 -> Add2/1, Add/1
  ic/1 -> Add2/2, Add/2
  Add/1 -> Gain1/1
  Gain/1 -> Add1/1
  Gain1/1 -> Add1/2
  Add1/1 -> ialpha/1
  Add2/1 -> Gain2/1
  Gain2/1 -> ibeta/1

== system foc/FOC_Model/currloop/Current_PI_Control ==
  id_fdbk : Inport  OutDataTypeStr=single
  iq_fdbk : Inport  Port=2  OutDataTypeStr=single
  id_ref : Inport  Port=3  OutDataTypeStr=single
  iq_ref : Inport  Port=4  OutDataTypeStr=single
  Constant3 : Constant  Value=Ls  OutDataTypeStr=single  SampleTime=-1
  Constant4 : Constant  Value=Rs  OutDataTypeStr=single  SampleTime=-1
  Gain : Gain  Gain=currt_width  OutDataTypeStr=single
  Gain1 : Gain  Gain=currt_width  OutDataTypeStr=single
  PID Controller : slpidlib/PID Controller  Controller=PI  Form=Parallel  TimeDomain=Discrete-time  UseExternalTs=off  SampleTime=-1  IntegratorMethod=Forward Euler  FilterMethod=Forward Euler  ControllerParametersSource=external  P=1  I=1  D=0  UseFilter=on  N=100  TunerSelectOption=Transfer Function Based (PID Tuner App)  InitialConditionSource=internal  InitialConditionForIntegrator=0  InitialConditionForFilter=0  DifferentiatorICPrevScaledInput=0  ExternalReset=none  TrackingMode=off  Kt=1  LimitOutput=on  SatLimitsSource=internal  UpperSaturationLimit=Ubus*0.9/sqrt(3)  LowerSaturationLimit=-Ubus*0.9/sqrt(3)  LinearizeAsGain=on  AntiWindupMode=none  Kb=1  POutMin=[]  POutMax=[]  IOutMin=[]  IOutMax=[]  DOutMin=[]  DOutMax=[]  NOutMin=[]  NOutMax=[]  SumOutMin=[]  SumOutMax=[]  SaturationOutMin=[]  SaturationOutMax=[]  PParamMin=[]  PParamMax=[]  IParamMin=[]  IParamMax=[]  DParamMin=[]  DParamMax=[]  NParamMin=[]  NParamMax=[]  KbParamMin=[]  KbParamMax=[]  KtParamMin=[]  KtParamMax=[]  KbOutMin=[]  KbOutMax=[]  KtOutMin=[]  KtOutMax=[]  IntegratorOutMin=[]  IntegratorOutMax=[]  FilterOutMin=[]  FilterOutMax=[]  SumI1OutMin=[]  SumI1OutMax=[]  SumI2OutMin=[]  SumI2OutMax=[]  SumI3OutMin=[]  SumI3OutMax=[]  SumI4OutMin=[]  SumI4OutMax=[]  SumDOutMin=[]  SumDOutMax=[]  DifferentiatorOutMin=[]  DifferentiatorOutMax=[]  FilterDiffOutCoefMin=[]  FilterDiffOutCoefMax=[]  ReciprocalOutMin=[]  ReciprocalOutMax=[]  SumDenOutMin=[]  SumDenOutMax=[]  SumNumOutMin=[]  SumNumOutMax=[]  DivideOutMin=[]  DivideOutMax=[]  UdiffTsProdOutMin=[]  UdiffTsProdOutMax=[]  NTsProdOutMin=[]  NTsProdOutMax=[]  UintegralTsProdOutMin=[]  UintegralTsProdOutMax=[]  UngainTsProdOutMin=[]  UngainTsProdOutMax=[]  IntegratorContinuousStateAttributes=''  IntegratorStateMustResolveToSignalObject=off  IntegratorRTWStateStorageClass=Auto  FilterContinuousStateAttributes=''  FilterStateMustResolveToSignalObject=off  FilterRTWStateStorageClass=Auto  ParallelPVariant=ExternalParameters  IdealPVariant=Disabled  IVariant=ExternalParameters  DVariant=Disabled  IntegratorVariant=Discrete  SatVariant=Enabled  AWVariant=Passthrough  PCopyVariant=Disabled  TRVariant=Disabled  FdbkBlocksVariant=Forward  IdealPFdbkVariant=Disabled  SatFdbkVariant=Disabled  DerivativeFilterVariant=Disabled  NVariant=Disabled  NCopyVariant=Disabled_SignalSpec  FilterICVariant=Disabled  IntegratorICVariant=InternalICs  ExternalResetVariant=Disabled  TRSumVariant=Passthrough  SumFdbkVariant=Disabled  SumVariant=Sum_PI  TsampFilterVariant=InternalTs  TsampNgainVariant=Passthrough  TsampIntegralVariant=Passthrough  ExternalSaturationOutDataTypeStr=Inherit: Same as second input
  PID Controller1 : slpidlib/PID Controller  Controller=PI  Form=Parallel  TimeDomain=Discrete-time  UseExternalTs=off  SampleTime=-1  IntegratorMethod=Forward Euler  FilterMethod=Forward Euler  ControllerParametersSource=external  P=1  I=1  D=0  UseFilter=on  N=100  TunerSelectOption=Transfer Function Based (PID Tuner App)  InitialConditionSource=internal  InitialConditionForIntegrator=0  InitialConditionForFilter=0  DifferentiatorICPrevScaledInput=0  ExternalReset=none  TrackingMode=off  Kt=1  LimitOutput=on  SatLimitsSource=internal  UpperSaturationLimit=Ubus*0.9/sqrt(3)  LowerSaturationLimit=-Ubus*0.9/sqrt(3)  LinearizeAsGain=on  AntiWindupMode=none  Kb=1  POutMin=[]  POutMax=[]  IOutMin=[]  IOutMax=[]  DOutMin=[]  DOutMax=[]  NOutMin=[]  NOutMax=[]  SumOutMin=[]  SumOutMax=[]  SaturationOutMin=[]  SaturationOutMax=[]  PParamMin=[]  PParamMax=[]  IParamMin=[]  IParamMax=[]  DParamMin=[]  DParamMax=[]  NParamMin=[]  NParamMax=[]  KbParamMin=[]  KbParamMax=[]  KtParamMin=[]  KtParamMax=[]  KbOutMin=[]  KbOutMax=[]  KtOutMin=[]  KtOutMax=[]  IntegratorOutMin=[]  IntegratorOutMax=[]  FilterOutMin=[]  FilterOutMax=[]  SumI1OutMin=[]  SumI1OutMax=[]  SumI2OutMin=[]  SumI2OutMax=[]  SumI3OutMin=[]  SumI3OutMax=[]  SumI4OutMin=[]  SumI4OutMax=[]  SumDOutMin=[]  SumDOutMax=[]  DifferentiatorOutMin=[]  DifferentiatorOutMax=[]  FilterDiffOutCoefMin=[]  FilterDiffOutCoefMax=[]  ReciprocalOutMin=[]  ReciprocalOutMax=[]  SumDenOutMin=[]  SumDenOutMax=[]  SumNumOutMin=[]  SumNumOutMax=[]  DivideOutMin=[]  DivideOutMax=[]  UdiffTsProdOutMin=[]  UdiffTsProdOutMax=[]  NTsProdOutMin=[]  NTsProdOutMax=[]  UintegralTsProdOutMin=[]  UintegralTsProdOutMax=[]  UngainTsProdOutMin=[]  UngainTsProdOutMax=[]  IntegratorContinuousStateAttributes=''  IntegratorStateMustResolveToSignalObject=off  IntegratorRTWStateStorageClass=Auto  FilterContinuousStateAttributes=''  FilterStateMustResolveToSignalObject=off  FilterRTWStateStorageClass=Auto  ParallelPVariant=ExternalParameters  IdealPVariant=Disabled  IVariant=ExternalParameters  DVariant=Disabled  IntegratorVariant=Discrete  SatVariant=Enabled  AWVariant=Passthrough  PCopyVariant=Disabled  TRVariant=Disabled  FdbkBlocksVariant=Forward  IdealPFdbkVariant=Disabled  SatFdbkVariant=Disabled  DerivativeFilterVariant=Disabled  NVariant=Disabled  NCopyVariant=Disabled_SignalSpec  FilterICVariant=Disabled  IntegratorICVariant=InternalICs  ExternalResetVariant=Disabled  TRSumVariant=Passthrough  SumFdbkVariant=Disabled  SumVariant=Sum_PI  TsampFilterVariant=InternalTs  TsampNgainVariant=Passthrough  TsampIntegralVariant=Passthrough  ExternalSaturationOutDataTypeStr=Inherit: Same as second input
  Sum1 : Sum  Inputs=|+-  AccumDataTypeStr=single  OutDataTypeStr=single
  Sum7 : Sum  Inputs=|+-  AccumDataTypeStr=single  OutDataTypeStr=single
  ud_ref : Outport  OutDataTypeStr=single
  uq_ref : Outport  Port=2  OutDataTypeStr=single
  wires:
  id_fdbk/1 -> Sum1/2
  id_ref/1 -> Sum1/1
  iq_fdbk/1 -> Sum7/2
  Sum1/1 -> PID Controller/1
  Sum7/1 -> PID Controller1/1
  PID Controller/1 -> ud_ref/1
  PID Controller1/1 -> uq_ref/1
  iq_ref/1 -> Sum7/1
  Constant4/1 -> Gain1/1
  Constant3/1 -> Gain/1
  Gain/1 -> PID Controller1/2, PID Controller/2
  Gain1/1 -> PID Controller1/3, PID Controller/3

== system foc/FOC_Model/currloop/Park_Trans ==
  note: id = ialpha*cos(theta)+ibeta*sin(theta);
      | iq = -ialpha*sin(theta)+ibeta*cos(theta);
  ialpha : Inport  OutDataTypeStr=single
  ibeta : Inport  Port=2  OutDataTypeStr=single
  theta : Inport  Port=3  OutDataTypeStr=single
  Add : Sum  AccumDataTypeStr=single  OutDataTypeStr=single
  Add1 : Sum  Inputs=-+  AccumDataTypeStr=single  OutDataTypeStr=single
  Cos : Trigonometry  Operator=cos  ApproximationMethod=Lookup
  Product{,1..3} (4 alike) : Product  OutDataTypeStr=single
  Sin : Trigonometry  ApproximationMethod=Lookup
  id : Outport  OutDataTypeStr=single
  iq : Outport  Port=2  OutDataTypeStr=single
  wires:
  ialpha/1 -> Product2/1, Product/1
  ibeta/1 -> Product3/1, Product1/1
  Product/1 -> Add/1
  Product1/1 -> Add/2
  Add/1 -> id/1
  Product2/1 -> Add1/1
  Product3/1 -> Add1/2
  Add1/1 -> iq/1
  theta/1 -> Cos/1, Sin/1
  Sin/1 -> Product1/2, Product2/2
  Cos/1 -> Product/2, Product3/2

== system foc/FOC_Model/currloop/SMO ==
  u_alpha : Inport  OutDataTypeStr=single
  u_beta : Inport  Port=2  OutDataTypeStr=single
  i_alpha : Inport  Port=3  OutDataTypeStr=single
  i_beta : Inport  Port=4  OutDataTypeStr=single
  PLL : Subsystem
  SMO : Subsystem
  Scope : Scope  NumInputPorts=2
  Scope1 : Scope  NumInputPorts=2
  theta : Outport
  we : Outport  Port=2
  tag scope: we_est=global
  wires:
  SMO/1(Ealpha^) -> PLL/1(e_alpha_est)
  SMO/2(Ebeta^) -> PLL/2(e_beta_est)
  u_alpha/1 -> Scope/1, SMO/1(u_alpha)
  i_alpha/1 -> Scope1/1, SMO/3(i_alpha)
  i_beta/1 -> Scope1/2, SMO/4(i_beta)
  PLL/1(theta_est) -> theta/1
  PLL/2(we_est) -> [we_est], we/1
  u_beta/1 -> Scope/2, SMO/2(u_beta)

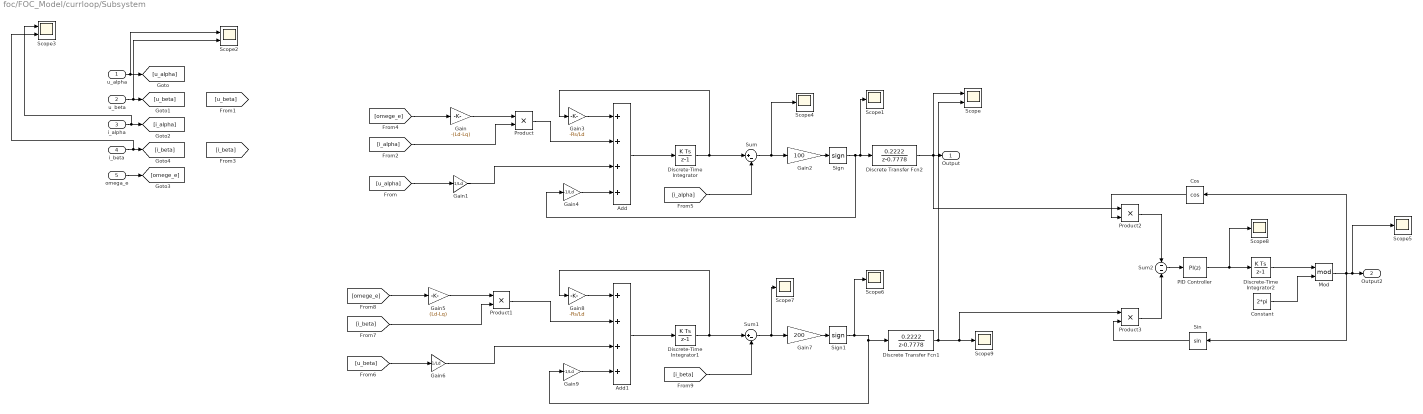
== system foc/FOC_Model/currloop/Subsystem ==
  u_alpha : Inport
  u_beta : Inport  Port=2
  i_alpha : Inport  Port=3
  i_beta : Inport  Port=4
  omega_e : Inport  Port=5
  Add : Sum  Inputs=++++
  Add1 : Sum  Inputs=++++
  Constant : Constant  Value=2*pi
  Cos : Trigonometry  Operator=cos
  Discrete Transfer Fcn1 : DiscreteTransferFcn  Numerator=[0.2222]  Denominator=[1 -0.7778]
  Discrete Transfer Fcn2 : DiscreteTransferFcn  Numerator=[0.2222]  Denominator=[1 -0.7778]
  Discrete-Time Integrator : DiscreteIntegrator  SampleTime=-1  ICPrevOutput=DiscIntNeverNeededParam  ICPrevScaledInput=DiscIntNeverNeededParam
  Discrete-Time Integrator1 : DiscreteIntegrator  SampleTime=-1  ICPrevOutput=DiscIntNeverNeededParam  ICPrevScaledInput=DiscIntNeverNeededParam
  Discrete-Time Integrator2 : DiscreteIntegrator  SampleTime=-1  ICPrevOutput=DiscIntNeverNeededParam  ICPrevScaledInput=DiscIntNeverNeededParam
  Gain : Gain  Gain=-(Ld-Lq)
  Gain1 : Gain  Gain=1/Ld
  Gain2 : Gain  Gain=100
  Gain3 : Gain  Gain=-Rs/Ld
  Gain4 : Gain  Gain=-1/Ld
  Gain5 : Gain  Gain=(Ld-Lq)
  Gain6 : Gain  Gain=1/Ld
  Gain7 : Gain  Gain=200
  Gain8 : Gain  Gain=-Rs/Ld
  Gain9 : Gain  Gain=-1/Ld
  Mod : Math  Operator=mod  SaturateOnIntegerOverflow=on
  PID Controller : slpidlib/PID Controller  Controller=PI  Form=Parallel  TimeDomain=Discrete-time  UseExternalTs=off  SampleTime=-1  IntegratorMethod=Forward Euler  FilterMethod=Forward Euler  ControllerParametersSource=internal  P=10  I=500  D=0  UseFilter=on  N=100  TunerSelectOption=Transfer Function Based (PID Tuner App)  InitialConditionSource=internal  InitialConditionForIntegrator=0  InitialConditionForFilter=0  DifferentiatorICPrevScaledInput=0  ExternalReset=none  TrackingMode=off  Kt=1  LimitOutput=off  SatLimitsSource=internal  UpperSaturationLimit=inf  LowerSaturationLimit=-inf  LinearizeAsGain=on  AntiWindupMode=none  Kb=1  POutMin=[]  POutMax=[]  IOutMin=[]  IOutMax=[]  DOutMin=[]  DOutMax=[]  NOutMin=[]  NOutMax=[]  SumOutMin=[]  SumOutMax=[]  SaturationOutMin=[]  SaturationOutMax=[]  PParamMin=[]  PParamMax=[]  IParamMin=[]  IParamMax=[]  DParamMin=[]  DParamMax=[]  NParamMin=[]  NParamMax=[]  KbParamMin=[]  KbParamMax=[]  KtParamMin=[]  KtParamMax=[]  KbOutMin=[]  KbOutMax=[]  KtOutMin=[]  KtOutMax=[]  IntegratorOutMin=[]  IntegratorOutMax=[]  FilterOutMin=[]  FilterOutMax=[]  SumI1OutMin=[]  SumI1OutMax=[]  SumI2OutMin=[]  SumI2OutMax=[]  SumI3OutMin=[]  SumI3OutMax=[]  SumI4OutMin=[]  SumI4OutMax=[]  SumDOutMin=[]  SumDOutMax=[]  DifferentiatorOutMin=[]  DifferentiatorOutMax=[]  FilterDiffOutCoefMin=[]  FilterDiffOutCoefMax=[]  ReciprocalOutMin=[]  ReciprocalOutMax=[]  SumDenOutMin=[]  SumDenOutMax=[]  SumNumOutMin=[]  SumNumOutMax=[]  DivideOutMin=[]  DivideOutMax=[]  UdiffTsProdOutMin=[]  UdiffTsProdOutMax=[]  NTsProdOutMin=[]  NTsProdOutMax=[]  UintegralTsProdOutMin=[]  UintegralTsProdOutMax=[]  UngainTsProdOutMin=[]  UngainTsProdOutMax=[]  IntegratorContinuousStateAttributes=''  IntegratorStateMustResolveToSignalObject=off  IntegratorRTWStateStorageClass=Auto  FilterContinuousStateAttributes=''  FilterStateMustResolveToSignalObject=off  FilterRTWStateStorageClass=Auto  ParallelPVariant=InternalParameters  IdealPVariant=Disabled  IVariant=InternalParameters  DVariant=Disabled  IntegratorVariant=Discrete  SatVariant=Disabled  AWVariant=Passthrough  PCopyVariant=Disabled  TRVariant=Disabled  FdbkBlocksVariant=Forward  IdealPFdbkVariant=Disabled  SatFdbkVariant=Disabled  DerivativeFilterVariant=Disabled  NVariant=Disabled  NCopyVariant=Disabled_SignalSpec  FilterICVariant=Disabled  IntegratorICVariant=InternalICs  ExternalResetVariant=Disabled  TRSumVariant=Passthrough  SumFdbkVariant=Disabled  SumVariant=Sum_PI  TsampFilterVariant=InternalTs  TsampNgainVariant=Passthrough  TsampIntegralVariant=Passthrough  ExternalSaturationOutDataTypeStr=Inherit: Same as second input
  Product{,1..3} (4 alike) : Product
  Scope : Scope  NumInputPorts=2
  Scope{1,4..9} (7 alike) : Scope
  Scope2 : Scope  NumInputPorts=2
  Scope3 : Scope  NumInputPorts=2
  Sign : Signum
  Sign1 : Signum
  Sin : Trigonometry
  Sum : Sum  Inputs=|+-
  Sum1 : Sum  Inputs=|+-
  Sum2 : Sum  Inputs=-|-
  Output : Outport
  Output2 : Outport  Port=2
  wires:
  u_alpha/1 -> Scope2/1, [u_alpha]
  u_beta/1 -> Scope2/2, [u_beta]
  i_alpha/1 -> Scope3/1, [i_alpha]
  i_beta/1 -> Scope3/2, [i_beta]
  omega_e/1 -> [omege_e]
  Gain/1 -> Product/1
  [omege_e] -> Gain/1
  [i_alpha] -> Product/2
  [u_alpha] -> Gain1/1
  Product/1 -> Add/2
  Gain1/1 -> Add/3
  Add/1 -> Discrete-Time Integrator/1
  Discrete-Time Integrator/1 -> Gain3/1, Sum/1
  [i_alpha] -> Sum/2
  Sum/1 -> Gain2/1, Scope4/1
  Gain3/1 -> Add/1
  Discrete Transfer Fcn2/1 -> Product2/1, Scope/1, Output/1
  Gain4/1 -> Add/4
  Product1/1 -> Add1/2
  Gain5/1 -> Product1/1
  [omege_e] -> Gain5/1
  Discrete-Time Integrator1/1 -> Gain8/1, Sum1/1
  Gain7/1 -> Sign1/1
  Add1/1 -> Discrete-Time Integrator1/1
  [i_beta] -> Product1/2
  [i_beta] -> Sum1/2
  [u_beta] -> Gain6/1
  Sign1/1 -> Scope6/1, Discrete Transfer Fcn1/1, Gain9/1
  Gain6/1 -> Add1/3
  Sum1/1 -> Scope7/1, Gain7/1
  Gain8/1 -> Add1/1
  Gain9/1 -> Add1/4
  PID Controller/1 -> Scope8/1, Discrete-Time Integrator2/1
  Discrete-Time Integrator2/1 -> Mod/1
  Constant/1 -> Mod/2
  Mod/1 -> Cos/1, Sin/1, Scope5/1, Output2/1
  Product2/1 -> Sum2/1
  Sum2/1 -> PID Controller/1
  Product3/1 -> Sum2/2
  Sin/1 -> Product3/2
  Cos/1 -> Product2/2
  Discrete Transfer Fcn1/1 -> Product3/1, Scope9/1, Scope/2
  Sign/1 -> Gain4/1, Scope1/1, Discrete Transfer Fcn2/1
  Gain2/1 -> Sign/1

== system foc/FOC_Model/currloop/observer ==
  Ualpha : Inport
  U_beta : Inport  Port=2
  Ialpha : Inport  Port=3
  Ibeta : Inport  Port=4
  Constant2 : Constant  Value=2*pi
  Data Type Conversion4 : DataTypeConversion  OutDataTypeStr=single
  Gain2 : Gain  Gain=Pn
  Mod1 : Math  Operator=mod  SaturateOnIntegerOverflow=on
  Scope5 : Scope  NumInputPorts=2
  fourth_SMO : Subsystem  TreatAsAtomicUnit=on
  wm->Nr2 : Gain  Gain=30/(pi*Pn)  OutDataTypeStr=single
  smo_theta : Outport
  smo_spd : Outport  Port=2
  wires:
  Ibeta/1 -> fourth_SMO/4(Ibeta)
  Data Type Conversion4/1 -> Mod1/2
  Ualpha/1 -> fourth_SMO/1(Ualpha)
  fourth_SMO/2(omega_e) -> wm->Nr2/1, Scope5/2
  fourth_SMO/1(Obe_Theta) -> Scope5/1, smo_theta/1
  Constant2/1 -> Data Type Conversion4/1
  Gain2/1 -> Mod1/1
  U_beta/1 -> fourth_SMO/2(U_beta)
  Ialpha/1 -> fourth_SMO/3(Ialpha)
  wm->Nr2/1 -> smo_spd/1  "real"

== system foc/FOC_Model/currloop/svpwm ==
  ud : Inport
  uq : Inport  Port=2
  Ubus : Inport  Port=3  SampleTime=0.0001
  theta : Inport  Port=4
  Anti_Park_Trans : Subsystem  TreatAsAtomicUnit=on
  Constant4 : Constant  Value=16000  OutDataTypeStr=single
  foc : MATLAB Function  TreatAsAtomicUnit=on
  Tcmp1 : Outport
  Tcmp2 : Outport  Port=2
  Tcmp3 : Outport  Port=3
  sector : Outport  Port=4
  tag scope: u_alpha=global, u_beta=global
  wires:
  foc/1(Tcmp1) -> Tcmp1/1
  Constant4/1 -> foc/4(Tpwm)
  Ubus/1 -> foc/3(Udc)
  uq/1 -> Anti_Park_Trans/2(uq)  "uq"
  foc/4(sector) -> sector/1
  ud/1 -> Anti_Park_Trans/1(ud)  "ud"
  foc/3(Tcmp3) -> Tcmp3/1
  foc/2(Tcmp2) -> Tcmp2/1
  theta/1 -> Anti_Park_Trans/3(theta)
  Anti_Park_Trans/1(ualpha) -> [u_alpha], foc/1(Valpha)  "u_alpha"
  Anti_Park_Trans/2(ubeta) -> [u_beta], foc/2(Vbeta)  "u_beta"

== system foc/FOC_Model/Motor_State/If Action Subsystem2/If Action Subsystem ==
  In1 : Inport
  Action Port : ActionPort
  delta_theta : Outport
  wires:
  In1/1 -> delta_theta/1

== system foc/FOC_Model/currloop/SMO/PLL ==
  e_alpha_est : Inport
  e_beta_est : Inport  Port=2
  Constant : Constant  Value=2*pi  SampleTime=-1
  Cos : Trigonometry  Operator=cos
  Discrete-Time Integrator : DiscreteIntegrator  SampleTime=-1  ICPrevOutput=DiscIntNeverNeededParam  ICPrevScaledInput=DiscIntNeverNeededParam
  IIR Filter : mcbcontrolslib/IIR Filter  VariantControl=Low Pass Filter  VariantSelect=Low-pass  Filter_constant=0.0004  advancedSettings=on  Ts=1e-6  cutOff_freq=63.6875
      settings: SourceProductBaseCode=MT
  IIR Filter1 : mcbcontrolslib/IIR Filter  VariantControl=Low Pass Filter  VariantSelect=Low-pass  Filter_constant=0.0004  advancedSettings=on  Ts=1e-5  cutOff_freq=6.3687
      settings: SourceProductBaseCode=MT
  Mod : Math  Operator=mod  SaturateOnIntegerOverflow=on
  PLL : Subsystem
      mask Display: disp('PI')
  Product : Product
  Product1 : Product
  Scope : Scope
  Sin : Trigonometry
  Sum : Sum  Inputs=--
  theta_est : Outport
  we_est : Outport  Port=2
  wires:
  e_alpha_est/1 -> Product/2
  Cos/1 -> Product/1
  Product/1 -> Sum/1
  e_beta_est/1 -> Product1/1
  Product1/1 -> Sum/2
  Sin/1 -> Product1/2
  Discrete-Time Integrator/1 -> Mod/1, Cos/1, Sin/1
  Sum/1 -> PLL/1(e)
  PLL/1(output) -> IIR Filter1/1, Discrete-Time Integrator/1
  IIR Filter1/1 -> Scope/1, we_est/1
  Mod/1 -> theta_est/1
  Constant/1 -> Mod/2

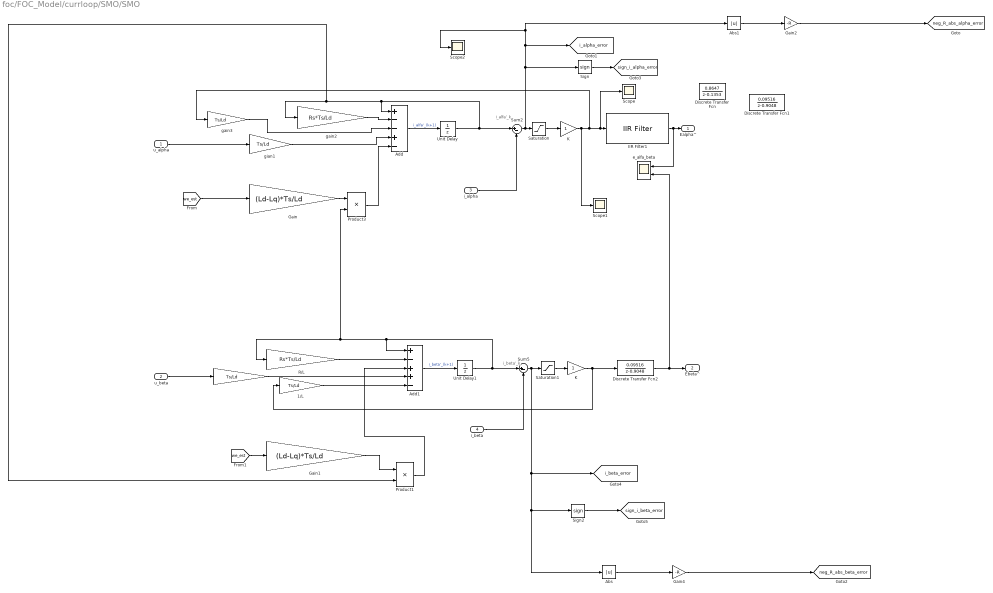
== system foc/FOC_Model/currloop/SMO/SMO ==
  note: i_alfa'_k
  note: i_beta'_k
  u_alpha : Inport  OutDataTypeStr=single
  u_beta : Inport  Port=2  OutDataTypeStr=single
  i_alpha : Inport  Port=3  OutDataTypeStr=single
  i_beta : Inport  Port=4  OutDataTypeStr=single
  " " : Gain  Gain=Ts/Ld
  " 1/L " : Gain  Gain=Ts/Ld
  Abs : Abs
  Abs1 : Abs
  Add : Sum  Inputs=+--+-  OutDataTypeStr=single
  Add1 : Sum  Inputs=+-++-
  Discrete Transfer Fcn : DiscreteTransferFcn  Numerator=[0.8647]  Denominator=[1 -0.1353]
  Discrete Transfer Fcn1 : DiscreteTransferFcn  Numerator=[0.09516]  Denominator=[1 -0.9048]
  Discrete Transfer Fcn2 : DiscreteTransferFcn  Numerator=[0.09516]  Denominator=[1 -0.9048]
  Gain : Gain  Gain=(Ld-Lq)*Ts/Ld
  Gain1 : Gain  Gain=(Ld-Lq)*Ts/Ld
  Gain2 : Gain  Gain=-R
  Gain4 : Gain  Gain=-R
  IIR Filter1 : mcbcontrolslib/IIR Filter  VariantControl=Low Pass Filter  VariantSelect=Low-pass  Filter_constant=0.1  advancedSettings=on  Ts=1e-4  cutOff_freq=176.8388
      settings: SourceProductBaseCode=MT
  K : Gain
  "K " : Gain
  Product1 : Product  RndMeth=Zero
  Product3 : Product  RndMeth=Zero
  "R/L " : Gain  Gain=Rs*Ts/Ld
  Saturation : Saturate  UpperLimit=2  LowerLimit=-2
  Saturation1 : Saturate  UpperLimit=2  LowerLimit=-2
  Scope : Scope
  Scope1 : Scope
  Scope2 : Scope
  Sign : Signum  ZeroCross=off
  Sign2 : Signum  ZeroCross=off
  Sum2 : Sum  Inputs=|+-
  Sum5 : Sum  Inputs=|+-
  Unit Delay : UnitDelay  SampleTime=-1  HasFrameUpgradeWarning=on
  Unit Delay1 : UnitDelay  SampleTime=-1  HasFrameUpgradeWarning=on
  e_alfa_beta : Scope  NumInputPorts=2
  gain2 : Gain  Gain=Rs*Ts/Ld  OutDataTypeStr=single
  gain3 : Gain  Gain=Ts/Ld
  gian1 : Gain  Gain=Ts/Ld
  Ealpha^ : Outport
  Ebeta^ : Outport  Port=2
  tag scope: i_alpha_error=global, i_beta_error=global, neg_R_abs_alpha_error=global, neg_R_abs_beta_error=global, sign_i_alpha_error=global, sign_i_beta_error=global
  wires:
  Saturation/1 -> K/1
  K/1 -> Scope1/1, IIR Filter1/1, Scope/1, gain3/1
  Unit Delay1/1 -> Add1/1, Product3/2, "R/L "/1, Sum5/1
  Saturation1/1 -> "K "/1
  " "/1 -> Add1/4
  "R/L "/1 -> Add1/2
  [we_est] -> Gain/1
  Gain/1 -> Product3/1
  Gain1/1 -> Product1/1
  [we_est] -> Gain1/1
  Product1/1 -> Add1/3
  Unit Delay/1 -> Product1/2, gain2/1, Add/1, Sum2/1
  Add/1 -> Unit Delay/1  "i_alfa'_(k+1)"
  gain2/1 -> Add/2
  gian1/1 -> Add/4
  Product3/1 -> Add/5
  gain3/1 -> Add/3
  Add1/1 -> Unit Delay1/1  "i_beta'_(k+1)"
  " 1/L "/1 -> Add1/5
  Sum2/1 -> Sign/1, [i_alpha_error], Scope2/1, Abs1/1, Saturation/1
  Gain2/1 -> [neg_R_abs_alpha_error]
  Abs1/1 -> Gain2/1
  Abs/1 -> Gain4/1
  Gain4/1 -> [neg_R_abs_beta_error]
  Sum5/1 -> Sign2/1, Abs/1, [i_beta_error], Saturation1/1
  Sign/1 -> [sign_i_alpha_error]
  Sign2/1 -> [sign_i_beta_error]
  u_alpha/1 -> gian1/1
  u_beta/1 -> " "/1
  i_alpha/1 -> Sum2/2
  i_beta/1 -> Sum5/2
  "K "/1 -> Discrete Transfer Fcn2/1, " 1/L "/1
  Discrete Transfer Fcn2/1 -> e_alfa_beta/2, Ebeta^/1
  IIR Filter1/1 -> e_alfa_beta/1, Ealpha^/1

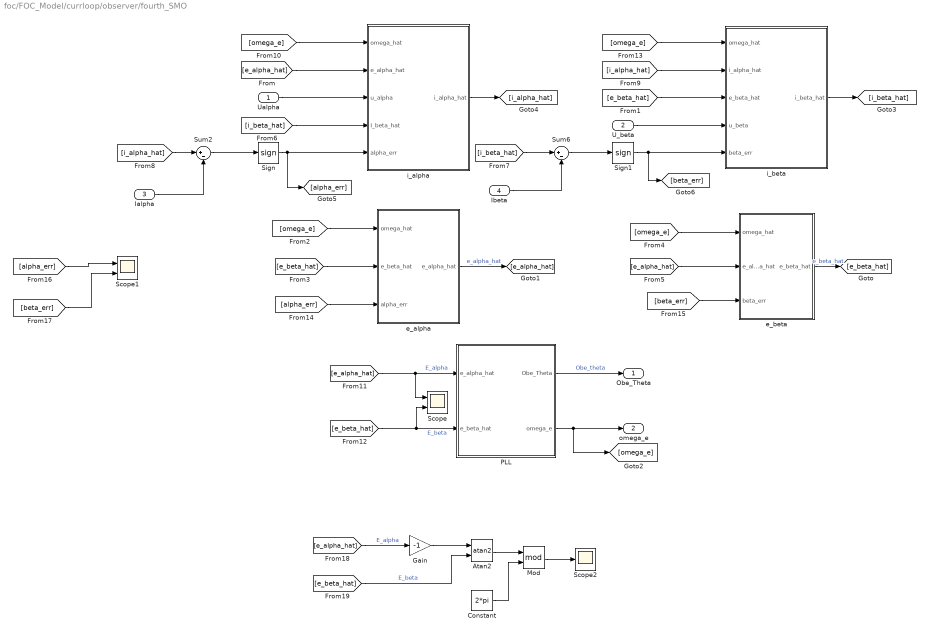
== system foc/FOC_Model/currloop/observer/fourth_SMO ==
  Ualpha : Inport
  U_beta : Inport  Port=2
  Ialpha : Inport  Port=3
  Ibeta : Inport  Port=4
  Atan2 : Trigonometry  Operator=atan2
  Constant : Constant  Value=2*pi  OutDataTypeStr=single
  Gain : Gain  Gain=-1  OutDataTypeStr=single
  Mod : Math  Operator=mod  SaturateOnIntegerOverflow=on
  PLL : Subsystem
  Scope : Scope  NumInputPorts=2
  Scope1 : Scope  NumInputPorts=2
  Scope2 : Scope
  Sign : Signum
  Sign1 : Signum
  Sum2 : Sum  Inputs=|+-
  Sum6 : Sum  Inputs=|+-
  e_alpha : Subsystem
  e_beta : Subsystem
  i_alpha : Subsystem
  i_beta : Subsystem
  Obe_Theta : Outport
  omega_e : Outport  Port=2
  wires:
  Sum6/1 -> Sign1/1
  Sum2/1 -> Sign/1
  Sign/1 -> i_alpha/5(alpha_err), [alpha_err]
  Ialpha/1 -> Sum2/2
  Sign1/1 -> [beta_err], i_beta/5(beta_err)
  Ibeta/1 -> Sum6/2
  i_alpha/1(i_alpha_hat) -> [i_alpha_hat]
  [e_alpha_hat] -> i_alpha/2(e_alpha_hat)
  Ualpha/1 -> i_alpha/3(u_alpha)
  [e_beta_hat] -> i_beta/3(e_beta_hat)
  U_beta/1 -> i_beta/4(u_beta)
  i_beta/1(i_beta_hat) -> [i_beta_hat]
  [i_beta_hat] -> i_alpha/4(I_beta_hat)
  [i_beta_hat] -> Sum6/1
  [i_alpha_hat] -> Sum2/1
  [i_alpha_hat] -> i_beta/2(i_alpha_hat)
  [omega_e] -> e_alpha/1(omega_hat)
  [e_beta_hat] -> e_alpha/2(e_beta_hat)
  [omega_e] -> e_beta/1(omega_hat)
  [e_alpha_hat] -> e_beta/2(e_alpha_hat)
  [omega_e] -> i_alpha/1(omega_hat)
  e_beta/1(e_beta_hat) -> [e_beta_hat]  "e_beta_hat"
  e_alpha/1(e_alpha_hat) -> [e_alpha_hat]  "e_alpha_hat"
  [e_alpha_hat] -> Scope/1, PLL/1(e_alpha_hat)  "E_alpha"
  [e_beta_hat] -> Scope/2, PLL/2(e_beta_hat)  "E_beta"
  PLL/2(omega_e) -> [omega_e], omega_e/1
  [omega_e] -> i_beta/1(omega_hat)
  PLL/1(Obe_Theta) -> Obe_Theta/1  "Obe_theta"
  [alpha_err] -> e_alpha/3(alpha_err)
  [beta_err] -> e_beta/3(beta_err)
  [alpha_err] -> Scope1/1
  [beta_err] -> Scope1/2
  [e_alpha_hat] -> Gain/1  "E_alpha"
  Gain/1 -> Atan2/1
  [e_beta_hat] -> Atan2/2  "E_beta"
  Atan2/1 -> Mod/1
  Constant/1 -> Mod/2
  Mod/1 -> Scope2/1

== system foc/FOC_Model/currloop/svpwm/Anti_Park_Trans ==
  note: Valpha = ud*cos(theta) - uq*sin(theta);
      | Vbeta = ud*sin(theta) + uq*cos(theta);
  ud : Inport  OutDataTypeStr=single
  uq : Inport  Port=2  OutDataTypeStr=single
  theta : Inport  Port=3
  Add : Sum  Inputs=+-
  Add1 : Sum
  Cos : Trigonometry  Operator=cos
  Product{,1..3} (4 alike) : Product
  Scope : Scope  NumInputPorts=2
  Sin : Trigonometry
  ualpha : Outport  OutDataTypeStr=single
  ubeta : Outport  Port=2  OutDataTypeStr=single
  wires:
  Add/1 -> ualpha/1
  ud/1 -> Product2/1, Product/1
  Cos/1 -> Product/2, Scope/2, Product3/2
  Product/1 -> Add/1
  uq/1 -> Product3/1, Product1/1
  theta/1 -> Sin/1, Cos/1
  Product1/1 -> Add/2
  Product2/1 -> Add1/1
  Product3/1 -> Add1/2
  Add1/1 -> ubeta/1
  Sin/1 -> Scope/1, Product2/2, Product1/2

== system foc/FOC_Model/currloop/SMO/PLL/PLL ==
  e : Inport
  Add : Sum
  Discrete-Time Integrator : DiscreteIntegrator  SampleTime=-1  ICPrevOutput=DiscIntNeverNeededParam  ICPrevScaledInput=DiscIntNeverNeededParam
  Ki : Gain  Gain=36000
  Kp : Gain  Gain=540
  Saturation : Saturate  UpperLimit=2000  LowerLimit=-2000
  output : Outport
  wires:
  Ki/1 -> Discrete-Time Integrator/1
  e/1 -> Kp/1, Ki/1
  Saturation/1 -> output/1
  Discrete-Time Integrator/1 -> Add/2
  Kp/1 -> Add/1
  Add/1 -> Saturation/1
